simulink model "CameraAngleCorrection"  (R2019b)
settings: Solver=VariableStepAuto  StartTime=0.0  StopTime=Inf  RelTol=1e-3
libraries: vrlib x4
settings Model: Creator=wul20  LastModifiedBy=z3527056
settings DataIOCC: LimitDataPoints=on  SaveOutput=off  SaveTime=off  ReturnWorkspaceOutputs=off
settings OptimizationCC: BlockReduction=off  BooleanDataType=off  LifeSpan=inf
settings DebuggingCC: SaveWithParameterizedLinksMsg=none  UnderspecifiedInitializationDetection=Classic  MergeDetectMultiDrivingBlocksExec=none  SignalResolutionControl=TryResolveAllWithWarning  AllowSymbolicDim=off  SFUnexpectedBacktrackingDiag=warning  SFNoUnconditionalDefaultTransitionDiag=warning  SFExecutionAtInitializationDiag=none  ArithmeticOperatorsInVariantConditions=warning
settings HardwareCC: TargetUnknown=on
settings SFSimCC: SimUseLocalCustomCode=off  CustomCodeUndefinedFunction=UseInterfaceOnly
settings RTWCC: RTWUseLocalCustomCode=off
settings CodeAppCC: StateflowObjectComments=on
settings GRTTargetCC: TargetLangStandard=C89/C90 (ANSI)  GeneratePreprocessorConditionals=Disable all

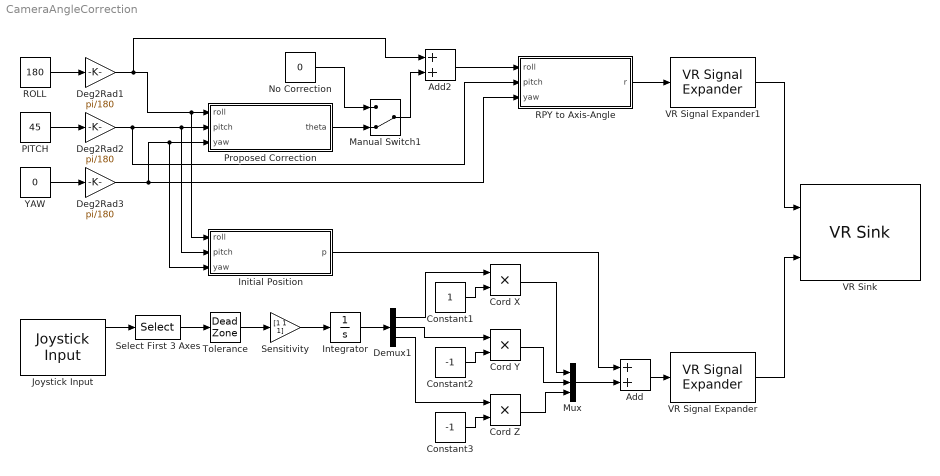
== system CameraAngleCorrection ==
  Add : Sum
  Add2 : Sum
  Constant1 : Constant
  Constant2 : Constant  Value=-1
  Constant3 : Constant  Value=-1
  Cord X : Product  Inputs=**
  Cord Y : Product  Inputs=**
  Cord Z : Product  Inputs=**
  Deg2Rad1 : Gain  Gain=pi/180
  Deg2Rad2 : Gain  Gain=pi/180
  Deg2Rad3 : Gain  Gain=pi/180
  Demux1 : Demux  Outputs=3
  Initial Position : MATLAB Function  TreatAsAtomicUnit=on
  Integrator : Integrator  InitialCondition=[0 0 0]  UpperSaturationLimit=[1000 1000 1000]  LowerSaturationLimit=[-1000 -1000 -1000]
  Joystick Input : vrlib/Joystick Input  joyid=1  adjustports=on  forcefeed=off
      settings: SourceProductBaseCode=VR
  Manual Switch1 : ManualSwitch  CurrentSetting=0
  Mux : Mux  Inputs=3
  No Correction : Constant  Value=0
  PITCH : Constant  Value=45
  Proposed Correction : MATLAB Function  TreatAsAtomicUnit=on
  ROLL : Constant  Value=180
  RPY to Axis-Angle : MATLAB Function  TreatAsAtomicUnit=on
  Select First 3 Axes : Selector  InputPortWidth=4  IndexOptions=Index vector (dialog)  Indices=[1 2 3]  OutputSizes=1
  "Sensitivity " : Gain  Gain=[1 1 1]
  Tolerance : DeadZone  LowerValue=[-0.1, -0.1, -0.5]  UpperValue=[0.1, 0.1, 0.5]  SaturateOnIntegerOverflow=on
  VR Signal Expander : vrlib/VR Signal Expander  outwidth=3  outidx=[1 2 3]
      settings: SourceProductName=Simulink 3D Animation  SourceProductBaseCode=VR
  VR Signal Expander1 : vrlib/VR Signal Expander  outwidth=4  outidx=[1 2 3 4]
      settings: SourceProductName=Simulink 3D Animation  SourceProductBaseCode=VR
  VR Sink : vrlib/VR Sink  InstantiateOnLoad=on  SampleTime=0.1  ViewEnable=on  RemoteChange=off  RemoteView=off  FieldsWritten=CameraGroup.rotation.4.1.1.double#CameraGroup.translation.3.1.1.double  WorldFileName=CameraAngleCorrection.wrl  AutoView=off  VideoDimensions=[]  AllowVariableSize=off
      settings: SourceProductBaseCode=VR
  YAW : Constant  Value=0
  wires:
  Joystick Input/1 -> Select First 3 Axes/1
  Select First 3 Axes/1 -> Tolerance/1
  "Sensitivity "/1 -> Integrator/1
  Constant1/1 -> Cord X/2
  Cord X/1 -> Mux/1
  Demux1/1 -> Cord X/1
  Demux1/2 -> Cord Y/1
  Demux1/3 -> Cord Z/1
  Constant3/1 -> Cord Z/2
  Constant2/1 -> Cord Y/2
  RPY to Axis-Angle/1(r) -> VR Signal Expander1/1
  PITCH/1 -> Deg2Rad2/1
  Add2/1 -> RPY to Axis-Angle/1(roll)
  Proposed Correction/1(theta) -> Manual Switch1/2
  No Correction/1 -> Manual Switch1/1
  Mux/1 -> Add/2
  Add/1 -> VR Signal Expander/1
  Cord Y/1 -> Mux/2
  Initial Position/1(p) -> Add/1
  VR Signal Expander1/1 -> VR Sink/1
  VR Signal Expander/1 -> VR Sink/2
  Deg2Rad1/1 -> Add2/1, Initial Position/1(roll), Proposed Correction/1(roll)
  Integrator/1 -> Demux1/1
  Tolerance/1 -> "Sensitivity "/1
  Deg2Rad2/1 -> Initial Position/2(pitch), Proposed Correction/2(pitch), RPY to Axis-Angle/2(pitch)
  ROLL/1 -> Deg2Rad1/1
  YAW/1 -> Deg2Rad3/1
  Deg2Rad3/1 -> RPY to Axis-Angle/3(yaw), Initial Position/3(yaw), Proposed Correction/3(yaw)
  Manual Switch1/1 -> Add2/2
  Cord Z/1 -> Mux/3

== matlab function CameraAngleCorrection/RPY to Axis-Angle ==
  data: roll input; r output; pitch input; yaw input
function r = CalRotation(roll, pitch, yaw)

DELTA=10^(-12);

R = roty(yaw)*rotx(pitch)*rotz(roll);

w = vlogR(R);

nw = norm(w);

if nw<DELTA
    
    r = [0; 0; 1; 0];
    
else

    r = [w/norm(w); norm(w)];

end

end

function [ w ] = vlogR( R )

DELTA=10^(-12);

tr=(trace(R)-1)/2;

if tr>1

    tr=1;

elseif tr<-1

    tr=-1;

end

phi=acos(tr);

if abs(phi)<DELTA

    w=[0;0;0];

elseif abs(phi-pi)<DELTA

    [V,D]=eig(R,'vector');

    D = real(D);
    
    V = real(V);
    
    if max(D)==D(1)
    
        w=V(:,1);
    
    elseif max(D)==D(2)
        
        w=V(:,2);
    
    else
        
        w=V(:,3);
    
    end
    
    if max(max(cos(phi)*eye(3)+(1-cos(phi))*(w*w')+sin(phi)*skew(w)-R))>DELTA
        
        w=-w;
    
    end
    
    w = w*phi;

else
    
    w=phi/(2*sin(phi))*[R(3,2)-R(2,3);R(1,3)-R(3,1);R(2,1)-R(1,2)];

end

end

== matlab function CameraAngleCorrection/Proposed Correction ==
  data: roll input; theta output; pitch input; yaw input
function theta = AngleCorrection(roll, pitch, yaw)

R = roty(yaw)*rotx(pitch)*rotz(roll);

x = R(1:3,1); y = R(1:3,2);

x0 = [1;0;0]; y0 = [0;1;0];

theta = FindNewAxes(x, y, x0, y0);

end


function theta = FindNewAxes(x, y, x0, y0)

theta = atan2(x0'*y-y0'*x,x0'*x+y0'*y);

end

== matlab function CameraAngleCorrection/Initial Position ==
  data: roll input; p output; pitch input; yaw input
function p = InitialPosition(roll, pitch, yaw)

R = roty(yaw)*rotx(pitch)*rotz(roll);

p = R*[30;30;140]+[0;0;-40];

end
